simulink library "AeroLib"  (Simulink 6.0)
settings: Solver=ode45  SolverMode=SingleTasking  StartTime=0.0  StopTime=10.0  RelTol=1e-3
undefined symbols (not defined in the file): Aero, Ap, Atm, Control, Controls, Eng, Flight_cg, Flight_DamperON, Flight_delta_isa, Flight_DeltaSpiral, Flight_InertiaSelect, Flight_ixx, Flight_ixz, Flight_iyy, Flight_izz, Flight_latitude, Flight_LoiterLenght, Flight_LoiterMode, Flight_LoiterRadius, Flight_longitude, Flight_MaxTargetPoints, Flight_SensorsON, Flight_TimeStep, Flight_TowerWind_X, Flight_TowerWind_Y, Flight_TowerWind_Z, Flight_TowerWindON, Flight_Trimming, Flight_TurbON, Flight_weight, Flight_WindGustON, Flight_WindShearON, Flight_ycg, Flight_zcg, Geom, Lgear, Mass, PEG_CDwbnp, PEG_CLht, PEG_CLht_elev, PEG_CLwbnp, PEG_CMht, PEG_CMwbnp, PEG_CNbeta, PEG_CNr, PEG_CNrud, PEG_CRail, PEG_CRbeta, PEG_CRp, PEG_CRrud, PEG_CYbeta, PEG_CYrud, pow, Sensors
libraries: AeroLib x133, simulink3 x49, simulink x37, aerospace x11
(part 5 of 7)

== system AeroLib/GroundReactions/Landing_Gear/GHM Ground_Reactions ==
  MUeLmg : Inport  Port=1  LatchInput=off
  MUsLmg : Inport  Port=2  LatchInput=off
  FstrLmg : Inport  Port=3  LatchInput=off
  Rlmg : Inport  Port=4  LatchInput=off
  TireCompLmg : Inport  Port=5  LatchInput=off
  MUeNg : Inport  Port=6  LatchInput=off
  MUsNg : Inport  Port=7  LatchInput=off
  FstrNg : Inport  Port=8  LatchInput=off
  Rng : Inport  Port=9  LatchInput=off
  TireCompNg : Inport  Port=10  LatchInput=off
  NoseWheelAng : Inport  Port=11  LatchInput=off
  EulerRad : Inport  Port=12  LatchInput=off
  MUeRmg : Inport  Port=13  LatchInput=off
  MUsRmg : Inport  Port=14  LatchInput=off
  FstrRmg : Inport  Port=15  LatchInput=off
  Rrmg : Inport  Port=16  LatchInput=off
  TireCompRmg : Inport  Port=17  LatchInput=off
  Bus Creator : BusCreator  DialogController=Simulink.DDGSource_Bus  Inputs=9
  Demux : Demux  Outputs=3
  Demux1 : Demux  Outputs=3
  Moments : Subsystem
  Reactions1 : Subsystem
  GR_Out : Outport
  wires:
  MUeLmg/1 -> Reactions1/1(MUeLmg)
  MUsLmg/1 -> Reactions1/2(MUsLmg)
  FstrLmg/1 -> Reactions1/3(FstrLmg)
  EulerRad/1 -> Reactions1/10(EulerRad)  "DCbg"
  MUeNg/1 -> Reactions1/4(MUeNg)
  MUsNg/1 -> Reactions1/5(MUsNg)
  FstrNg/1 -> Reactions1/6(FstrNg)
  MUeRmg/1 -> Reactions1/7(MUeRmg)
  MUsRmg/1 -> Reactions1/8(MUsRmg)
  FstrRmg/1 -> Reactions1/9(FstrRmg)
  Reactions1/2(FgearLMG) -> Moments/1(FgearLmg)
  Reactions1/3(FgearNG) -> Moments/2(FgearNg)
  Reactions1/4(FgearRMG) -> Moments/3(FgearRmg)
  Rlmg/1 -> Moments/4(Rlmg)
  TireCompLmg/1 -> Bus Creator/7  "TireCompLmg"
  Rng/1 -> Moments/5(Rng)
  TireCompNg/1 -> Bus Creator/8  "TireCompNg"
  Rrmg/1 -> Moments/6(Rrmg)
  TireCompRmg/1 -> Bus Creator/9  "TireCompRmg"
  NoseWheelAng/1 -> Reactions1/11(NoseWheelAng)
  Bus Creator/1 -> GR_Out/1
  Reactions1/1(Fgear) -> Demux/1
  Demux/1 -> Bus Creator/1  "Xground"
  Demux/2 -> Bus Creator/2  "Yground"
  Demux/3 -> Bus Creator/3  "Zground"
  Moments/1(Mgear) -> Demux1/1
  Demux1/1 -> Bus Creator/4  "Lground"
  Demux1/2 -> Bus Creator/5  "Mground"
  Demux1/3 -> Bus Creator/6  "Nground"

== system AeroLib/GroundReactions/Landing_Gear/Left Main Gear Dynamics ==
  Brake : Inport  Port=1  LatchInput=off
  VelB : Inport  Port=2  LatchInput=off
  RatesB : Inport  Port=3  LatchInput=off
  DCbg : Inport  Port=4  LatchInput=off
  Hagl : Inport  Port=5  LatchInput=off
  Conf_Tire_RposLmg : Inport  Port=6  LatchInput=off
  Ground_Tire Contact : Subsystem
  Ground_Tire Friction : Subsystem
  LGEAR Accelerations : Subsystem
  LGEAR States : Subsystem
  MUeff : Outport
  MUside : Outport  Port=2
  TireForce : Outport  Port=3
  Rtb : Outport  Port=4
  TireComp : Outport  Port=5
  wires:
  Conf_Tire_RposLmg/1 -> Ground_Tire Contact/7(Conf_Tire_RposLmg)
  DCbg/1 -> Ground_Tire Contact/1(DCbg)
  Brake/1 -> Ground_Tire Friction/3(Brake)
  Ground_Tire Contact/2(Vtg) -> Ground_Tire Friction/2(Vtg)
  Ground_Tire Contact/1(Rtb) -> Rtb/1
  VelB/1 -> Ground_Tire Contact/2(VelB)
  RatesB/1 -> Ground_Tire Contact/3(RatesB)
  Ground_Tire Friction/2(MUeff) -> MUeff/1
  Ground_Tire Friction/1(MUside) -> MUside/1
  LGEAR States/1(Sdot) -> Ground_Tire Contact/4(Sdot), LGEAR Accelerations/2(Sdot)
  LGEAR States/2(S) -> Ground_Tire Contact/5(S), LGEAR Accelerations/3(S)
  LGEAR Accelerations/2(S2dot) -> LGEAR States/1(S2dot)
  LGEAR Accelerations/3(TireComp) -> Ground_Tire Contact/6(TireComp), TireComp/1
  Hagl/1 -> LGEAR Accelerations/1(Hagl)
  LGEAR Accelerations/1(TireForce) -> Ground_Tire Friction/1(TireForce), TireForce/1

== system AeroLib/GroundReactions/Landing_Gear/Nose Gear Dynamics ==
  VelB : Inport  Port=1  LatchInput=off
  RatesB : Inport  Port=2  LatchInput=off
  DCbg : Inport  Port=3  LatchInput=off
  Hagl : Inport  Port=4  LatchInput=off
  Conf_Tire_RposNg : Inport  Port=5  LatchInput=off
  Caster : Inport  Port=6  LatchInput=off
  NoseWheel : Inport  Port=7  LatchInput=off
  Ground_Tire Contact : Subsystem
  Ground_Tire Friction : Subsystem
  LGEAR Accelerations : Subsystem
  LGEAR States : Subsystem
  NoseWheelAngle : Subsystem
  MUeff : Outport
  MUside : Outport  Port=2
  TireForce : Outport  Port=3
  Rtb : Outport  Port=4
  TireComp : Outport  Port=5
  NoseWheelAng : Outport  Port=6
  wires:
  Conf_Tire_RposNg/1 -> Ground_Tire Contact/7(Conf_Tire_RposNg)
  LGEAR Accelerations/1(TireForce) -> TireForce/1, Ground_Tire Friction/1(TireForce)
  Hagl/1 -> LGEAR Accelerations/1(Hagl)
  LGEAR Accelerations/3(TireComp) -> Ground_Tire Contact/6(TireComp), TireComp/1
  LGEAR Accelerations/2(S2dot) -> LGEAR States/1(S2dot)
  LGEAR States/2(S) -> Ground_Tire Contact/5(S), LGEAR Accelerations/3(S)
  LGEAR States/1(Sdot) -> Ground_Tire Contact/4(Sdot), LGEAR Accelerations/2(Sdot)
  Ground_Tire Friction/1(MUside) -> MUside/1
  Ground_Tire Friction/2(MUeff) -> MUeff/1
  RatesB/1 -> Ground_Tire Contact/3(RatesB)
  VelB/1 -> Ground_Tire Contact/2(VelB)
  Ground_Tire Contact/1(Rtb) -> Rtb/1
  Ground_Tire Contact/2(Vtg) -> Ground_Tire Friction/2(Vtg), NoseWheelAngle/1(Vtg)
  DCbg/1 -> Ground_Tire Contact/1(DCbg)
  Caster/1 -> NoseWheelAngle/2(Caster)
  NoseWheel/1 -> NoseWheelAngle/3(NoseWheelAng)
  NoseWheelAngle/1(Out1) -> NoseWheelAng/1

== system AeroLib/GroundReactions/Landing_Gear/Right Main Gear Dynamics ==
  Brake : Inport  Port=1  LatchInput=off
  VelB : Inport  Port=2  LatchInput=off
  RatesB : Inport  Port=3  LatchInput=off
  DCbg : Inport  Port=4  LatchInput=off
  Hagl : Inport  Port=5  LatchInput=off
  Conf_Tire_RposRmg : Inport  Port=6  LatchInput=off
  Ground_Tire Contact : Subsystem
  Ground_Tire Friction : Subsystem
  LGEAR Accelerations : Subsystem
  LGEAR States : Subsystem
  MUeff : Outport
  MUside : Outport  Port=2
  TireForce : Outport  Port=3
  Rtb : Outport  Port=4
  TireComp : Outport  Port=5
  wires:
  LGEAR Accelerations/3(TireComp) -> TireComp/1, Ground_Tire Contact/6(TireComp)
  LGEAR Accelerations/2(S2dot) -> LGEAR States/1(S2dot)
  Conf_Tire_RposRmg/1 -> Ground_Tire Contact/7(Conf_Tire_RposRmg)
  DCbg/1 -> Ground_Tire Contact/1(DCbg)
  Brake/1 -> Ground_Tire Friction/3(Brake)
  Ground_Tire Contact/2(Vtg) -> Ground_Tire Friction/2(Vtg)
  Ground_Tire Contact/1(Rtb) -> Rtb/1
  VelB/1 -> Ground_Tire Contact/2(VelB)
  RatesB/1 -> Ground_Tire Contact/3(RatesB)
  Ground_Tire Friction/2(MUeff) -> MUeff/1
  Ground_Tire Friction/1(MUside) -> MUside/1
  LGEAR States/1(Sdot) -> LGEAR Accelerations/2(Sdot), Ground_Tire Contact/4(Sdot)
  LGEAR States/2(S) -> LGEAR Accelerations/3(S), Ground_Tire Contact/5(S)
  Hagl/1 -> LGEAR Accelerations/1(Hagl)
  LGEAR Accelerations/1(TireForce) -> Ground_Tire Friction/1(TireForce), TireForce/1

== system AeroLib/Propulsion/Booster/Fthrust_Booster ==
  LH NT : Inport  Port=1  LatchInput=off
  Constant : Constant  Value=0
  Fcn : Fcn  Expr=u*cos(pitch*pi/180)
  Fcn2 : Fcn  Expr=-u*sin(pitch*pi/180)
  Mux : Mux  Inputs=3
  LHFthr : Outport
  wires:
  Mux/1 -> LHFthr/1
  Fcn2/1 -> Mux/3
  Constant/1 -> Mux/2
  Fcn/1 -> Mux/1
  LH NT/1 -> Fcn/1, Fcn2/1

== system AeroLib/Propulsion/Booster/Thrust ==
  In1 : Inport  Port=1  LatchInput=off
  From_Reset : Inport  Port=2  LatchInput=off
  Constant : Constant  Value=0
  Gain_Amp : Gain  Gain=10  SaturateOnIntegerOverflow=on
  Stateless_Integrator : AeroLib/AMS_StatelessFilters/Stateless_Integrator
  Sum : Sum  Inputs=|+-  SaturateOnIntegerOverflow=on  InputSameDT=on
  Out1 : Outport
  wires:
  Sum/1 -> Gain_Amp/1  "err"
  Stateless_Integrator/1 -> Sum/2, Out1/1  "Stab"
  Gain_Amp/1 -> Stateless_Integrator/3
  In1/1 -> Sum/1
  Constant/1 -> Stateless_Integrator/2
  From_Reset/1 -> Stateless_Integrator/1

== system AeroLib/Propulsion/Engine_Transient/Engine_Transient_LH ==
  Throttle : Inport  Port=1  LatchInput=off
  From_Reset : Inport  Port=2  LatchInput=off
  Max : Constant  Value=Eng.MaxThrottle
  Min : Constant  Value=Eng.MinThrottle
  SpoolUpFreq : Gain  Gain=0.02  SaturateOnIntegerOverflow=on
  Stateless_LimIntegrator : AeroLib/AMS_StatelessFilters/Stateless_LimIntegrator
  Sum : Sum  Inputs=|+-  SaturateOnIntegerOverflow=on  InputSameDT=on
  TLA : Outport
  wires:
  SpoolUpFreq/1 -> Stateless_LimIntegrator/3
  Sum/1 -> SpoolUpFreq/1
  Stateless_LimIntegrator/1 -> Sum/2, TLA/1
  Throttle/1 -> Sum/1, Stateless_LimIntegrator/2
  Max/1 -> Stateless_LimIntegrator/5
  Min/1 -> Stateless_LimIntegrator/4
  From_Reset/1 -> Stateless_LimIntegrator/1

== system AeroLib/Propulsion/Engine_Transient/Engine_Transient_RH ==
  Throttle : Inport  Port=1  LatchInput=off
  From_Reset : Inport  Port=2  LatchInput=off
  Max : Constant  Value=Eng.MaxThrottle
  Min : Constant  Value=Eng.MinThrottle
  SpoolUpFreq : Gain  Gain=0.02  SaturateOnIntegerOverflow=on
  Stateless_LimIntegrator : AeroLib/AMS_StatelessFilters/Stateless_LimIntegrator
  Sum : Sum  Inputs=|+-  SaturateOnIntegerOverflow=on  InputSameDT=on
  TLA : Outport
  wires:
  From_Reset/1 -> Stateless_LimIntegrator/1
  Min/1 -> Stateless_LimIntegrator/4
  Max/1 -> Stateless_LimIntegrator/5
  Throttle/1 -> Stateless_LimIntegrator/2, Sum/1
  Stateless_LimIntegrator/1 -> TLA/1, Sum/2
  Sum/1 -> SpoolUpFreq/1
  SpoolUpFreq/1 -> Stateless_LimIntegrator/3

== system AeroLib/Propulsion/Fixed_Pitch_Propeller/Mach_Number_Effect ==
  J : Inport  Port=1  LatchInput=off
  Prop_rps : Inport  Port=2  LatchInput=off
  TAS : Inport  Port=3  LatchInput=off
  Mach : Inport  Port=4  LatchInput=off
  CP_coef : simulink/Lookup Tables/Interpolation (n-D) using PreLookup  numDimsPopupSelect=2  explicitNumDims=2  table=Eng.Prop.Kcp'  interpMethod=Linear  extrapMethod=Linear  rangeErrorMode=None  NumSelectionDims=0
  Constant : Constant  Value=0.75*pi
  Constant1 : Constant  Value=Eng.Prop.Twist
  Gain2 : Gain  Gain=180/pi  SaturateOnIntegerOverflow=on
  Km_coef : simulink/Lookup Tables/Interpolation (n-D) using PreLookup  numDimsPopupSelect=2  explicitNumDims=2  table=Eng.Prop.Kct'  interpMethod=Linear  extrapMethod=Linear  rangeErrorMode=None  NumSelectionDims=0
  Mach_Propeller : Fcn  Expr=sqrt( u(2)^2 + (pi*u(1)*Eng.Prop.diam)^2)/u(3)
  Mux2 : Mux  Inputs=3
  PreLook-Up Index Search : simulink/Lookup Tables/PreLookup Index Search  bpData=Eng.Prop.alp  searchMode=Binary Search  cacheBpFlag=off  outputFlag=off  IndexDataType=uint32  extrapMode=Linear Extrapolation  rangeErrorMode=None
  PreLook-Up Index Search1 : simulink/Lookup Tables/PreLookup Index Search  bpData=Eng.Prop.Mr  searchMode=Binary Search  cacheBpFlag=off  outputFlag=off  IndexDataType=uint32  extrapMode=Linear Extrapolation  rangeErrorMode=None
  Product2 : Product  Inputs=*/  SaturateOnIntegerOverflow=on  InputSameDT=on
  Product3 : Product  Inputs=*/  SaturateOnIntegerOverflow=on  InputSameDT=on
  Saturation : Saturate  UpperLimit=1.7  LowerLimit=1
  Saturation1 : Saturate  UpperLimit=1  LowerLimit=0.8
  Sum : Sum  Inputs=|-+  SaturateOnIntegerOverflow=on  InputSameDT=on
  Trigonometric Function : Trigonometry  Operator=atan
  Km : Outport
  Kcp : Outport  Port=2
  wires:
  Mux2/1 -> Mach_Propeller/1
  Product2/1 -> Mux2/3
  CP_coef/1 -> Saturation/1
  Sum/1 -> PreLook-Up Index Search/1
  Constant1/1 -> Sum/2
  Gain2/1 -> Sum/1
  Mach_Propeller/1 -> PreLook-Up Index Search1/1
  PreLook-Up Index Search/1 -> CP_coef/2, Km_coef/2
  PreLook-Up Index Search1/1 -> CP_coef/1, Km_coef/1
  Trigonometric Function/1 -> Gain2/1
  Product3/1 -> Trigonometric Function/1
  Constant/1 -> Product3/2
  Prop_rps/1 -> Mux2/1
  TAS/1 -> Mux2/2, Product2/1
  J/1 -> Product3/1
  Saturation/1 -> Kcp/1
  Mach/1 -> Product2/2
  Km_coef/1 -> Saturation1/1
  Saturation1/1 -> Km/1

== system AeroLib/Propulsion/Jet_Engine/Engine_Tables ==
  TRA : Inport  Port=1  LatchInput=off
  Mach : Inport  Port=2  LatchInput=off
  Alt : Inport  Port=3  LatchInput=off
  From_Reset : Inport  Port=4  LatchInput=off
  FuelCut : Inport  Port=5  LatchInput=off
  Constant1 : Constant  Value=0
  Constant5 : Constant  Value=0
  Constant6 : Constant  Value=Eng.Fuel.mass
  Fcn1 : Fcn  Expr=u(2)*(1-u(1))
  Fcn2 : Fcn  Expr=u(1)*(1-u(2))
  Fcn3 : Fcn  Expr=1-u
  FuelDensity : Gain  Gain=0.7  SaturateOnIntegerOverflow=on
  Fuel_Flow : simulink/Lookup Tables/Interpolation (n-D) using PreLookup  numDimsPopupSelect=1  explicitNumDims=2  table=Eng.Cons  interpMethod=Linear  extrapMethod=Linear  rangeErrorMode=None  NumSelectionDims=0
  Gross_Thrust : simulink/Lookup Tables/Interpolation (n-D) using PreLookup  numDimsPopupSelect=3  explicitNumDims=2  table=Eng.GrossThrust  interpMethod=Linear  extrapMethod=Linear  rangeErrorMode=None  NumSelectionDims=0
  Mux : Mux  Inputs=2
  Mux1 : Mux  Inputs=2
  PreLook-Up Index Search : simulink/Lookup Tables/PreLookup Index Search  bpData=Eng.Mach  searchMode=Binary Search  cacheBpFlag=off  outputFlag=off  IndexDataType=uint32  extrapMode=Linear Extrapolation  rangeErrorMode=None
  PreLook-Up Index Search1 : simulink/Lookup Tables/PreLookup Index Search  bpData=Eng.Alt  searchMode=Binary Search  cacheBpFlag=off  outputFlag=off  IndexDataType=uint32  extrapMode=Linear Extrapolation  rangeErrorMode=None
  PreLook-Up Index Search2 : simulink/Lookup Tables/PreLookup Index Search  bpData=Eng.Throttle  searchMode=Binary Search  cacheBpFlag=off  outputFlag=off  IndexDataType=uint32  extrapMode=Linear Extrapolation  rangeErrorMode=None
  Product : Product  SaturateOnIntegerOverflow=on  InputSameDT=on
  Ram_Drag : simulink/Lookup Tables/Interpolation (n-D) using PreLookup  numDimsPopupSelect=3  explicitNumDims=2  table=Eng.RamDrag  interpMethod=Linear  extrapMethod=Linear  rangeErrorMode=None  NumSelectionDims=0
  Stateless_LimIntegrator : AeroLib/AMS_StatelessFilters/Stateless_LimIntegrator
  Sum1 : Sum  Inputs=+-  SaturateOnIntegerOverflow=on  InputSameDT=on
  GrossThrust : Outport
  NetThrust : Outport  Port=2
  RamDrag : Outport  Port=3
  Fuel_Mass : Outport  Port=4
  wires:
  Fuel_Flow/1 -> Product/1
  Product/1 -> FuelDensity/1
  Fcn3/1 -> Product/2
  Sum1/1 -> NetThrust/1  "NetThrust"
  Alt/1 -> PreLook-Up Index Search1/1
  Mach/1 -> PreLook-Up Index Search/1
  TRA/1 -> PreLook-Up Index Search2/1
  Ram_Drag/1 -> Mux/2  "RamDrag"
  PreLook-Up Index Search2/1 -> Fuel_Flow/1, Ram_Drag/1, Gross_Thrust/1
  PreLook-Up Index Search1/1 -> Ram_Drag/3, Gross_Thrust/3
  PreLook-Up Index Search/1 -> Ram_Drag/2, Gross_Thrust/2
  Fcn1/1 -> RamDrag/1, Sum1/2  "RamDrag"
  FuelCut/1 -> Fcn3/1, Mux/1, Mux1/2
  Mux/1 -> Fcn1/1
  Fcn2/1 -> GrossThrust/1, Sum1/1  "GrossThrust"
  Gross_Thrust/1 -> Mux1/1  "GrossThrust"
  Mux1/1 -> Fcn2/1
  FuelDensity/1 -> Stateless_LimIntegrator/3
  Constant1/1 -> Stateless_LimIntegrator/2
  From_Reset/1 -> Stateless_LimIntegrator/1
  Constant5/1 -> Stateless_LimIntegrator/4
  Constant6/1 -> Stateless_LimIntegrator/5
  Stateless_LimIntegrator/1 -> Fuel_Mass/1

== system AeroLib/Propulsion/Piston_Engine_Propeller/Power_Limit ==
  Avail_Power : Inport  Port=1  LatchInput=off
  Rpm : Inport  Port=2  LatchInput=off
  Power_Demand : Inport  Port=3  LatchInput=off
  Fcn1 : Fcn  Expr=u >= 0
  Fcn2 : Fcn  Expr=u(1) - u(2)
  Fcn4 : Fcn  Expr=u < 0
  Gain : Gain  Orientation=left  Gain=5  SaturateOnIntegerOverflow=on
  Memory2 : Memory  Orientation=left
  Mux1 : Mux  Inputs=2
  Product1 : Product  SaturateOnIntegerOverflow=on  InputSameDT=on
  Rpm_Limit : Subsystem
  Sum1 : Sum  Orientation=left  Inputs=+++  SaturateOnIntegerOverflow=on  InputSameDT=on
  Switch : Switch  Threshold=0.5  SaturateOnIntegerOverflow=on  InputSameDT=on
  Delta_Rpm : Outport  Orientation=left
  wires:
  Gain/1 -> Delta_Rpm/1
  Switch/1 -> Sum1/3
  Rpm_Limit/1(Rpm_Command) -> Sum1/2
  Rpm/1 -> Rpm_Limit/2(Rpm)
  Power_Demand/1 -> Mux1/2
  Avail_Power/1 -> Mux1/1
  Product1/1 -> Switch/1
  Fcn4/1 -> Product1/1
  Memory2/1 -> Gain/1, Fcn4/1, Sum1/1
  Sum1/1 -> Memory2/1
  Mux1/1 -> Fcn2/1
  Fcn1/1 -> Switch/2
  Fcn2/1 -> Rpm_Limit/1(deltaPower), Switch/3, Product1/2, Fcn1/1

== system AeroLib/Propulsion/Thrust_Components/LH_Fthrust ==
  LH NT : Inport  Port=1  LatchInput=off
  Fcn : Fcn  Expr=u*cos(pitch)*cos(toeout)
  Fcn1 : Fcn  Expr=-u*sin(toeout)
  Fcn2 : Fcn  Expr=-u*sin(pitch)
  Mux : Mux  Inputs=3
  LHFthr : Outport
  wires:
  Mux/1 -> LHFthr/1
  Fcn2/1 -> Mux/3
  Fcn1/1 -> Mux/2
  Fcn/1 -> Mux/1
  LH NT/1 -> Fcn2/1, Fcn1/1, Fcn/1

== system AeroLib/Propulsion/Thrust_Components/RH_Fthrust ==
  RH NT : Inport  Port=1  LatchInput=off
  Fcn : Fcn  Expr=u*cos(pitch)*cos(toeout)
  Fcn1 : Fcn  Expr=u*sin(toeout)
  Fcn2 : Fcn  Expr=-u*sin(pitch)
  Mux : Mux  Inputs=3
  RHFthr : Outport
  wires:
  RH NT/1 -> Fcn/1, Fcn1/1, Fcn2/1
  Fcn/1 -> Mux/1
  Fcn1/1 -> Mux/2
  Fcn2/1 -> Mux/3
  Mux/1 -> RHFthr/1

== system AeroLib/Propulsion/Variable_Pitch_Propeller/Mach_Number_Effect ==
  J : Inport  Port=1  LatchInput=off
  Prop_rps : Inport  Port=2  LatchInput=off
  TAS : Inport  Port=3  LatchInput=off
  Mach : Inport  Port=4  LatchInput=off
  Prop_Pitch_deg : Inport  Port=5  LatchInput=off
  CP_coef : simulink/Lookup Tables/Interpolation (n-D) using PreLookup  numDimsPopupSelect=2  explicitNumDims=2  table=Eng.Prop.Kcp'  interpMethod=Linear  extrapMethod=Linear  rangeErrorMode=None  NumSelectionDims=0
  Constant : Constant  Value=0.75*pi
  Gain2 : Gain  Gain=180/pi  SaturateOnIntegerOverflow=on
  Km_coef : simulink/Lookup Tables/Interpolation (n-D) using PreLookup  numDimsPopupSelect=2  explicitNumDims=2  table=Eng.Prop.Kct'  interpMethod=Linear  extrapMethod=Linear  rangeErrorMode=None  NumSelectionDims=0
  Mach_Propeller : Fcn  Expr=sqrt( u(2)^2 + (pi*u(1)*Eng.Prop.diam)^2)/u(3)
  Mux2 : Mux  Inputs=3
  PreLook-Up Index Search : simulink/Lookup Tables/PreLookup Index Search  bpData=Eng.Prop.alp  searchMode=Binary Search  cacheBpFlag=off  outputFlag=off  IndexDataType=uint32  extrapMode=Linear Extrapolation  rangeErrorMode=None
  PreLook-Up Index Search1 : simulink/Lookup Tables/PreLookup Index Search  bpData=Eng.Prop.Mr  searchMode=Binary Search  cacheBpFlag=off  outputFlag=off  IndexDataType=uint32  extrapMode=Linear Extrapolation  rangeErrorMode=None
  Product2 : Product  Inputs=*/  SaturateOnIntegerOverflow=on  InputSameDT=on
  Product3 : Product  Inputs=*/  SaturateOnIntegerOverflow=on  InputSameDT=on
  Saturation : Saturate  UpperLimit=1.7  LowerLimit=1
  Saturation1 : Saturate  UpperLimit=1  LowerLimit=0.8
  Sum : Sum  Inputs=|-+  SaturateOnIntegerOverflow=on  InputSameDT=on
  Trigonometric Function : Trigonometry  Operator=atan
  Km : Outport
  Kcp : Outport  Port=2
  wires:
  Mux2/1 -> Mach_Propeller/1
  Product2/1 -> Mux2/3
  CP_coef/1 -> Saturation/1
  Sum/1 -> PreLook-Up Index Search/1
  Prop_Pitch_deg/1 -> Sum/2
  Gain2/1 -> Sum/1
  Mach_Propeller/1 -> PreLook-Up Index Search1/1
  PreLook-Up Index Search/1 -> CP_coef/2, Km_coef/2
  PreLook-Up Index Search1/1 -> CP_coef/1, Km_coef/1
  Trigonometric Function/1 -> Gain2/1
  Product3/1 -> Trigonometric Function/1
  Constant/1 -> Product3/2
  Prop_rps/1 -> Mux2/1
  TAS/1 -> Mux2/2, Product2/1
  J/1 -> Product3/1
  Saturation/1 -> Kcp/1
  Mach/1 -> Product2/2
  Km_coef/1 -> Saturation1/1
  Saturation1/1 -> Km/1

== system AeroLib/Sensors/Air_Data_Computer/SensorsOFF ==
  Clock : Clock
      settings: Decimation=10
  Constant1 : Constant  Value=Flight_SensorsON
  Fcn : Fcn  Expr=u <= 0+eps
  or : Logic  Operator=OR
  or1 : Logic  Operator=NOT
  SensorsOFF : Outport
  wires:
  Clock/1 -> Fcn/1
  Constant1/1 -> or1/1  "DT"
  Fcn/1 -> or/2
  or/1 -> SensorsOFF/1
  or1/1 -> or/1

== system AeroLib/Sensors/Global_Positioning_System/SensorsOFF ==
  Clock : Clock
      settings: Decimation=10
  Constant1 : Constant  Value=Flight_SensorsON
  Fcn : Fcn  Expr=u <= 0+eps
  or : Logic  Operator=OR
  or1 : Logic  Operator=NOT
  SensorsOFF : Outport
  wires:
  or1/1 -> or/1
  or/1 -> SensorsOFF/1
  Fcn/1 -> or/2
  Constant1/1 -> or1/1  "DT"
  Clock/1 -> Fcn/1

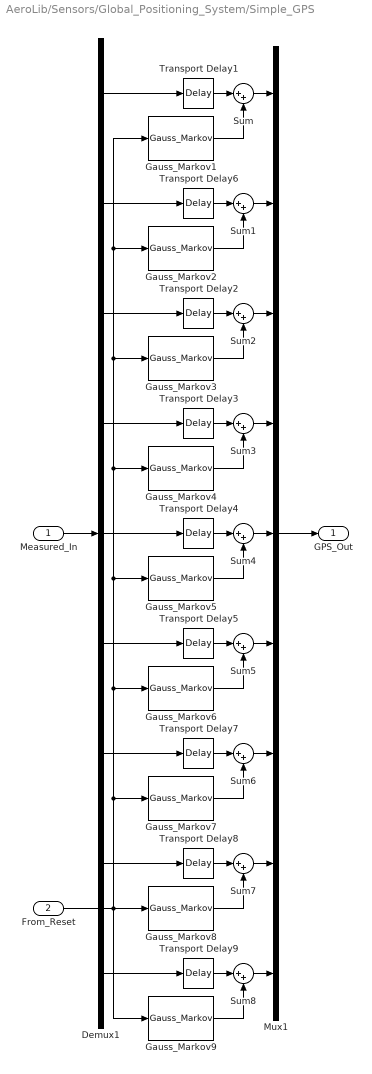
== system AeroLib/Sensors/Global_Positioning_System/Simple_GPS ==
  Measured_In : Inport  Port=1  LatchInput=off
  "From_Reset " : Inport  Port=2  LatchInput=off
  Demux1 : Demux  Outputs=9
  Gauss_Markov1 : AeroLib/Sensors/Gauss_Markov  Seed=Seed(1)  tau=Time(1)  Var=Var(1)
  Gauss_Markov2 : AeroLib/Sensors/Gauss_Markov  Seed=Seed(2)  tau=Time(2)  Var=Var(2)
  Gauss_Markov3 : AeroLib/Sensors/Gauss_Markov  Seed=Seed(3)  tau=Time(3)  Var=Var(3)
  Gauss_Markov4 : AeroLib/Sensors/Gauss_Markov  Seed=Seed(4)  tau=Time(4)  Var=Var(4)
  Gauss_Markov5 : AeroLib/Sensors/Gauss_Markov  Seed=Seed(5)  tau=Time(5)  Var=Var(5)
  Gauss_Markov6 : AeroLib/Sensors/Gauss_Markov  Seed=Seed(6)  tau=Time(6)  Var=Var(6)
  Gauss_Markov7 : AeroLib/Sensors/Gauss_Markov  Seed=Seed(7)  tau=Time(7)  Var=Var(7)
  Gauss_Markov8 : AeroLib/Sensors/Gauss_Markov  Seed=Seed(8)  tau=Time(8)  Var=Var(8)
  Gauss_Markov9 : AeroLib/Sensors/Gauss_Markov  Seed=Seed(9)  tau=Time(9)  Var=Var(9)
  Mux1 : Mux  Inputs=9
  Sum{,1..8} (9 alike) : Sum  Inputs=|++  SaturateOnIntegerOverflow=on  InputSameDT=on
  Transport Delay1 : TransportDelay  DelayTime=Time_delay(1)
  Transport Delay2 : TransportDelay  DelayTime=Time_delay(3)
  Transport Delay3 : TransportDelay  DelayTime=Time_delay(4)
  Transport Delay4 : TransportDelay  DelayTime=Time_delay(5)
  Transport Delay5 : TransportDelay  DelayTime=Time_delay(6)
  Transport Delay6 : TransportDelay  DelayTime=Time_delay(2)
  Transport Delay7 : TransportDelay  DelayTime=Time_delay(7)
  Transport Delay8 : TransportDelay  DelayTime=Time_delay(8)
  Transport Delay9 : TransportDelay  DelayTime=Time_delay(9)
  GPS_Out : Outport
  wires:
  Mux1/1 -> GPS_Out/1
  Measured_In/1 -> Demux1/1
  Gauss_Markov1/1 -> Sum/2
  Transport Delay1/1 -> Sum/1
  Gauss_Markov2/1 -> Sum1/2
  Transport Delay6/1 -> Sum1/1
  Gauss_Markov3/1 -> Sum2/2
  Transport Delay2/1 -> Sum2/1
  Gauss_Markov4/1 -> Sum3/2
  Transport Delay3/1 -> Sum3/1
  Gauss_Markov5/1 -> Sum4/2
  Transport Delay4/1 -> Sum4/1
  Demux1/2 -> Transport Delay6/1
  Demux1/3 -> Transport Delay2/1
  Sum1/1 -> Mux1/2
  Demux1/4 -> Transport Delay3/1
  Sum3/1 -> Mux1/4
  Sum4/1 -> Mux1/5
  Demux1/5 -> Transport Delay4/1
  Gauss_Markov6/1 -> Sum5/2
  Transport Delay5/1 -> Sum5/1
  Sum5/1 -> Mux1/6
  Demux1/6 -> Transport Delay5/1
  Sum2/1 -> Mux1/3
  Demux1/1 -> Transport Delay1/1
  Sum/1 -> Mux1/1
  Gauss_Markov7/1 -> Sum6/2
  Transport Delay7/1 -> Sum6/1
  Sum6/1 -> Mux1/7
  Demux1/7 -> Transport Delay7/1
  Gauss_Markov8/1 -> Sum7/2
  Transport Delay8/1 -> Sum7/1
  Sum7/1 -> Mux1/8
  Demux1/8 -> Transport Delay8/1
  "From_Reset "/1 -> Gauss_Markov9/1, Gauss_Markov7/1, Gauss_Markov6/1, Gauss_Markov5/1, Gauss_Markov4/1, Gauss_Markov3/1, Gauss_Markov2/1, Gauss_Markov1/1, Gauss_Markov8/1
  Gauss_Markov9/1 -> Sum8/2
  Transport Delay9/1 -> Sum8/1
  Demux1/9 -> Transport Delay9/1
  Sum8/1 -> Mux1/9

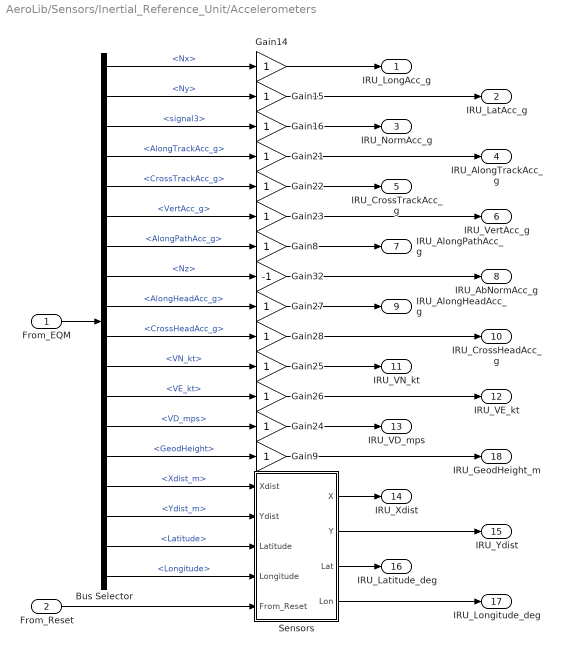
== system AeroLib/Sensors/Inertial_Reference_Unit/Accelerometers ==
  From_EQM : Inport  Port=1  LatchInput=off
  From_Reset : Inport  Port=2  LatchInput=off
  Bus Selector : BusSelector  DialogController=Simulink.DDGSource_Bus  OutputSignals=Nx,Ny,AccB.signal3,AlongTrackAcc_g,CrossTrackAcc_g,VertAcc_g,AlongPathAcc_g,Nz,AlongHeadAcc_g,CrossHeadAcc_g,VN_kt,VE_kt,VD_mps,GeodHeight,Xdist_m,Ydist_m,Latitude,Longitude
  Gain{8..9,14..16,21..28} (13 alike) : Gain  SaturateOnIntegerOverflow=on
  Gain32 : Gain  Gain=-1  SaturateOnIntegerOverflow=on
  Sensors : Subsystem
  IRU_LongAcc_g : Outport
  IRU_LatAcc_g : Outport  Port=2
  IRU_NormAcc_g : Outport  Port=3
  IRU_AlongTrackAcc_g : Outport  Port=4
  IRU_CrossTrackAcc_g : Outport  Port=5
  IRU_VertAcc_g : Outport  Port=6
  IRU_AlongPathAcc_g : Outport  Port=7
  IRU_AbNormAcc_g : Outport  Port=8
  IRU_AlongHeadAcc_g : Outport  Port=9
  IRU_CrossHeadAcc_g : Outport  Port=10
  IRU_VN_kt : Outport  Port=11
  IRU_VE_kt : Outport  Port=12
  IRU_VD_mps : Outport  Port=13
  IRU_Xdist : Outport  Port=14
  IRU_Ydist : Outport  Port=15
  IRU_Latitude_deg : Outport  Port=16
  IRU_Longitude_deg : Outport  Port=17
  IRU_GeodHeight_m : Outport  Port=18
  wires:
  From_Reset/1 -> Sensors/5(From_Reset)
  Bus Selector/14 -> Gain9/1  "<GeodHeight>"
  Gain9/1 -> IRU_GeodHeight_m/1
  Bus Selector/18 -> Sensors/4(Longitude)  "<Longitude>"
  Sensors/4(Lon) -> IRU_Longitude_deg/1
  Sensors/3(Lat) -> IRU_Latitude_deg/1
  Bus Selector/16 -> Sensors/2(Ydist)  "<Ydist_m>"
  Bus Selector/15 -> Sensors/1(Xdist)  "<Xdist_m>"
  Bus Selector/17 -> Sensors/3(Latitude)  "<Latitude>"
  Sensors/1(X) -> IRU_Xdist/1
  Sensors/2(Y) -> IRU_Ydist/1
  Bus Selector/13 -> Gain24/1  "<VD_mps>"
  Bus Selector/12 -> Gain26/1  "<VE_kt>"
  Bus Selector/11 -> Gain25/1  "<VN_kt>"
  Bus Selector/10 -> Gain28/1  "<CrossHeadAcc_g>"
  Bus Selector/9 -> Gain27/1  "<AlongHeadAcc_g>"
  Bus Selector/8 -> Gain32/1  "<Nz>"
  Bus Selector/7 -> Gain8/1  "<AlongPathAcc_g>"
  Bus Selector/6 -> Gain23/1  "<VertAcc_g>"
  Bus Selector/5 -> Gain22/1  "<CrossTrackAcc_g>"
  Bus Selector/4 -> Gain21/1  "<AlongTrackAcc_g>"
  Bus Selector/3 -> Gain16/1  "<signal3>"
  Bus Selector/2 -> Gain15/1  "<Ny>"
  Bus Selector/1 -> Gain14/1  "<Nx>"
  Gain24/1 -> IRU_VD_mps/1
  Gain25/1 -> IRU_VN_kt/1
  Gain26/1 -> IRU_VE_kt/1
  Gain27/1 -> IRU_AlongHeadAcc_g/1
  Gain28/1 -> IRU_CrossHeadAcc_g/1
  Gain32/1 -> IRU_AbNormAcc_g/1
  Gain8/1 -> IRU_AlongPathAcc_g/1
  Gain23/1 -> IRU_VertAcc_g/1
  Gain21/1 -> IRU_AlongTrackAcc_g/1
  Gain22/1 -> IRU_CrossTrackAcc_g/1
  Gain14/1 -> IRU_LongAcc_g/1
  Gain15/1 -> IRU_LatAcc_g/1
  Gain16/1 -> IRU_NormAcc_g/1
  From_EQM/1 -> Bus Selector/1

== system AeroLib/Sensors/Inertial_Reference_Unit/Airspeed_Detectors ==
  From_EQM : Inport  Port=1  LatchInput=off
  From_Atmos : Inport  Port=2  LatchInput=off
  From_Reset : Inport  Port=3  LatchInput=off
  Bus Selector : BusSelector  DialogController=Simulink.DDGSource_Bus  OutputSignals=GroundSpeed_kt
  Bus Selector1 : BusSelector  DialogController=Simulink.DDGSource_Bus  OutputSignals=KIAS,TAS_kt
  Constant : Constant
  Demux : Demux  Outputs=3
  MinMax : MinMax  Function=max  Inputs=2  SaturateOnIntegerOverflow=on  InputSameDT=on
  Mux : Mux  Inputs=3
  SensorsOFF : Subsystem
  Simple_Sensor : AeroLib/Sensors/Simple_Sensor  Var=Sensors.IRU.Speed.Var  Seed=Sensors.IRU.Speed.Seed  Max=600  Min=0  Time_Const=Sensors.IRU.Speed.TimeConst
  Switch : Switch  Threshold=0.5  SaturateOnIntegerOverflow=on  InputSameDT=on
  IRU_GrSpeed_kt : Outport
  IRU_KIAS : Outport  Port=2
  IRU_TAS_kt : Outport  Port=3
  wires:
  Simple_Sensor/1 -> Switch/3
  From_Reset/1 -> Simple_Sensor/3
  Mux/1 -> Simple_Sensor/2, Switch/1, Simple_Sensor/1
  Demux/2 -> IRU_KIAS/1
  Demux/3 -> IRU_TAS_kt/1
  SensorsOFF/1(SensorsOFF) -> Switch/2
  Bus Selector1/2 -> Mux/3  "<TAS_kt>"
  Bus Selector1/1 -> Mux/2  "<KIAS>"
  Bus Selector/1 -> Mux/1  "<GroundSpeed_kt>"
  From_Atmos/1 -> Bus Selector1/1
  From_EQM/1 -> Bus Selector/1
  Demux/1 -> IRU_GrSpeed_kt/1
  Switch/1 -> MinMax/2
  MinMax/1 -> Demux/1
  Constant/1 -> MinMax/1

== system AeroLib/Sensors/Inertial_Reference_Unit/Altitude_Sensors ==
  From_Atmos : Inport  Port=1  LatchInput=off
  From_EQM : Inport  Port=2  LatchInput=off
  From_Reset : Inport  Port=3  LatchInput=off
  Bus Selector1 : BusSelector  DialogController=Simulink.DDGSource_Bus  OutputSignals=PresAlt_ft
  Bus Selector2 : BusSelector  DialogController=Simulink.DDGSource_Bus  OutputSignals=Hagl_ft
  SensorsOFF : Subsystem
  Simple_Sensor : AeroLib/Sensors/Simple_Sensor  Var=Sensors.IRU.Alt.Pres.Var  Seed=Sensors.IRU.Alt.Pres.Seed  Max=60000  Min=-500  Time_Const=Sensors.IRU.Alt.Pres.TimeConst
  Simple_Sensor1 : AeroLib/Sensors/Simple_Sensor  Var=Sensors.IRU.Alt.Radar.Var  Seed=Sensors.IRU.Alt.Radar.Seed  Max=3000  Min=0  Time_Const=Sensors.IRU.Alt.Radar.TimeConst
  Switch : Switch  Threshold=0.5  SaturateOnIntegerOverflow=on  InputSameDT=on
  Switch1 : Switch  Threshold=0.5  SaturateOnIntegerOverflow=on  InputSameDT=on
  IRU_PresAlt_ft : Outport
  IRU_RadarAlt_ft : Outport  Port=2
  wires:
  From_Reset/1 -> Simple_Sensor1/3, Simple_Sensor/3
  Simple_Sensor1/1 -> Switch1/3
  Simple_Sensor/1 -> Switch/3
  SensorsOFF/1(SensorsOFF) -> Switch1/2, Switch/2
  Bus Selector2/1 -> Simple_Sensor1/2, Switch1/1, Simple_Sensor1/1  "<Hagl_ft>"
  From_EQM/1 -> Bus Selector2/1
  From_Atmos/1 -> Bus Selector1/1
  Bus Selector1/1 -> Simple_Sensor/2, Switch/1, Simple_Sensor/1  "<PresAlt_ft>"
  Switch/1 -> IRU_PresAlt_ft/1
  Switch1/1 -> IRU_RadarAlt_ft/1

== system AeroLib/Sensors/Inertial_Reference_Unit/Flow_Incidence_Angle_Sensors ==
  From_Atmos : Inport  Port=1  LatchInput=off
  From_Reset : Inport  Port=2  LatchInput=off
  Bus Selector1 : BusSelector  DialogController=Simulink.DDGSource_Bus  OutputSignals=Alpha,Beta
  Demux : Demux  Outputs=2
  Mux : Mux  Inputs=2
  SensorsOFF : Subsystem
  Simple_Sensor : AeroLib/Sensors/Simple_Sensor  Var=Sensors.IRU.AlphaBeta.Var  Seed=Sensors.IRU.AlphaBeta.Seed  Max=30  Min=-30  Time_Const=Sensors.IRU.AlphaBeta.TimeConst
  Switch : Switch  Threshold=0.5  SaturateOnIntegerOverflow=on  InputSameDT=on
  IRU_Alpha : Outport
  IRU_Beta : Outport  Port=2
  wires:
  Simple_Sensor/1 -> Switch/3
  From_Reset/1 -> Simple_Sensor/3
  Mux/1 -> Simple_Sensor/2, Switch/1, Simple_Sensor/1
  Switch/1 -> Demux/1
  Demux/2 -> IRU_Beta/1
  Demux/1 -> IRU_Alpha/1
  SensorsOFF/1(SensorsOFF) -> Switch/2
  Bus Selector1/2 -> Mux/2  "<Beta>"
  Bus Selector1/1 -> Mux/1  "<Alpha>"
  From_Atmos/1 -> Bus Selector1/1

== system AeroLib/Sensors/Inertial_Reference_Unit/Gyrospopes ==
  From_EQM : Inport  Port=1  LatchInput=off
  Bus Selector : BusSelector  DialogController=Simulink.DDGSource_Bus  OutputSignals=Phi_deg,The_deg,P_deg,Q_deg,R_deg,Track_deg,Psi_deg,Gamma_deg
  Fcn : Fcn  Expr=u+MagDev
  Fcn1 : Fcn  Expr=u+MagDev
  Fcn2 : Fcn  Expr=u+PlatformDev
  Gain{3..7,9..10} (7 alike) : Gain  SaturateOnIntegerOverflow=on
  Pitch_Gyro : Gain  SaturateOnIntegerOverflow=on
  Pitch_Rate_Gyro : Gain  SaturateOnIntegerOverflow=on
  Roll_Gyro : Gain  SaturateOnIntegerOverflow=on
  Roll_Rate_Gyro : Gain  SaturateOnIntegerOverflow=on
  Sum : Sum  Inputs=+-|  SaturateOnIntegerOverflow=on  InputSameDT=on
  Yaw_Rate_Gyro : Gain  SaturateOnIntegerOverflow=on
  IRU_Theta_deg : Outport
  IRU_Phi_deg : Outport  Port=2
  IRU_Q_degps : Outport  Port=3
  IRU_P_degps : Outport  Port=4
  IRU_R_degps : Outport  Port=5
  IRU_Track_deg : Outport  Port=6
  IRU_Head_deg : Outport  Port=7
  IRU_TrackMag_deg : Outport  Port=8
  IRU_HeadMag_deg : Outport  Port=9
  IRU_DriftAngle_deg : Outport  Port=10
  IRU_PlatformHead_deg : Outport  Port=11
  IRU_FPath_deg : Outport  Port=12
  wires:
  Gain10/1 -> IRU_FPath_deg/1
  Gain9/1 -> IRU_PlatformHead_deg/1
  Gain7/1 -> IRU_DriftAngle_deg/1
  Gain6/1 -> IRU_HeadMag_deg/1
  Gain5/1 -> IRU_TrackMag_deg/1
  Gain4/1 -> IRU_Head_deg/1
  Gain3/1 -> IRU_Track_deg/1
  Bus Selector/6 -> Fcn/1, Gain3/1, Sum/1  "<Track_deg>"
  Bus Selector/8 -> Gain10/1  "<Gamma_deg>"
  Bus Selector/7 -> Fcn1/1, Gain4/1, Sum/2, Fcn2/1  "<Psi_deg>"
  Fcn/1 -> Gain5/1
  Fcn1/1 -> Gain6/1
  Sum/1 -> Gain7/1
  Fcn2/1 -> Gain9/1
  Bus Selector/4 -> Pitch_Rate_Gyro/1  "<Q_deg>"
  Pitch_Gyro/1 -> IRU_Theta_deg/1
  Roll_Gyro/1 -> IRU_Phi_deg/1
  Pitch_Rate_Gyro/1 -> IRU_Q_degps/1
  Roll_Rate_Gyro/1 -> IRU_P_degps/1
  Yaw_Rate_Gyro/1 -> IRU_R_degps/1
  Bus Selector/2 -> Pitch_Gyro/1  "<The_deg>"
  Bus Selector/1 -> Roll_Gyro/1  "<Phi_deg>"
  Bus Selector/3 -> Roll_Rate_Gyro/1  "<P_deg>"
  Bus Selector/5 -> Yaw_Rate_Gyro/1  "<R_deg>"
  From_EQM/1 -> Bus Selector/1

== system AeroLib/Aerodynamics/Aerodynamics_Generic/LIft/CL Tail ==
  From_Inputs : Inport  Port=1  LatchInput=off
  Epsilon : Inport  Port=2  LatchInput=off
  From_Atmos : Inport  Port=3  LatchInput=off
  From_EQM : Inport  Port=4  LatchInput=off
  Bus Selector : BusSelector  DialogController=Simulink.DDGSource_Bus  OutputSignals=Elev_deg,Stab_deg
  Bus Selector1 : BusSelector  DialogController=Simulink.DDGSource_Bus  OutputSignals=Alpha,TAS,AlphaDot
  Bus Selector2 : BusSelector  DialogController=Simulink.DDGSource_Bus  OutputSignals=Q_rad
  Fcn1 : Fcn  Expr=u(1)+u(2)-u(3)+u(4)
  Fcn3 : Fcn  Expr=Geom.Htail.lt/u(1)*180/pi*(1.2*u(3)+0.32*u(2))
  Fcn5 : Fcn  Expr=(Aero.a1_deg*u(2) )*Geom.Htail.st/Geom.Wing.sw
  Fcn6 : Fcn  Expr=( Aero.a2_deg*u(1))*Geom.Htail.st/Geom.Wing.sw
  Gain : Gain  Gain=PEG_CLht  SaturateOnIntegerOverflow=on
  Gain1 : Gain  Gain=PEG_CLht_elev  SaturateOnIntegerOverflow=on
  Mux : Mux  Inputs=3
  Mux1 : Mux
  Mux2 : Mux  Inputs=2
  Sum : Sum  Inputs=|++  SaturateOnIntegerOverflow=on  InputSameDT=on
  CL_Tail : Outport
  wires:
  Gain1/1 -> Sum/2
  Gain/1 -> Sum/1
  Fcn6/1 -> Gain1/1
  Fcn5/1 -> Gain/1  "CL_Tail"
  Sum/1 -> CL_Tail/1
  Bus Selector/1 -> Mux2/1  "<Elev_deg>"
  Fcn3/1 -> Mux1/4
  Bus Selector1/3 -> Mux/2  "<AlphaDot>"
  From_Inputs/1 -> Bus Selector/1
  From_Atmos/1 -> Bus Selector1/1
  From_EQM/1 -> Bus Selector2/1
  Bus Selector1/1 -> Mux1/2  "<Alpha>"
  Bus Selector1/2 -> Mux/1  "<TAS>"
  Bus Selector/2 -> Mux1/1  "<Stab_deg>"
  Bus Selector2/1 -> Mux/3  "<Q_rad>"
  Mux/1 -> Fcn3/1
  Fcn1/1 -> Mux2/2  "alpha_ht"
  Mux1/1 -> Fcn1/1
  Mux2/1 -> Fcn6/1, Fcn5/1
  Epsilon/1 -> Mux1/3  "Epsilon"

== system AeroLib/Aerodynamics/Aerodynamics_Pioneer/Aero Total/Stab2Body ==
  Alpha_Deg : Inport  Port=1  LatchInput=off
  Stab_Axis : Inport  Port=2  LatchInput=off
  Constant{1..2,4..5} (4 alike) : Constant  Value=0
  Constant3 : Constant
  Deg-->Rad : Gain  Gain=pi/180  SaturateOnIntegerOverflow=on
  Deg-->Rad1 : Gain  Gain=-1  SaturateOnIntegerOverflow=on
  Deg-->Rad2 : Gain  Gain=-1  SaturateOnIntegerOverflow=on
  Deg-->Rad3 : Gain  Gain=-1  SaturateOnIntegerOverflow=on
  Mux : Mux  Inputs=9
  Product : Product  Multiplication=Matrix(*)  SaturateOnIntegerOverflow=on  InputSameDT=on
  Reshape : simulink3/Signals & Systems/Reshape  OutputDimensionality=Customize  OutputDimensions=[3,3]
  Trigonometric Function : Trigonometry  Operator=cos
  Trigonometric Function2 : Trigonometry
  Trigonometric Function3 : Trigonometry  Operator=cos
  Trigonometric Function4 : Trigonometry
  Body_Axis : Outport
  wires:
  Deg-->Rad2/1 -> Mux/3
  Deg-->Rad3/1 -> Mux/9
  Deg-->Rad1/1 -> Mux/1
  Trigonometric Function3/1 -> Deg-->Rad3/1
  Constant4/1 -> Mux/8
  Trigonometric Function4/1 -> Mux/7
  Constant1/1 -> Mux/6
  Constant3/1 -> Mux/5
  Constant5/1 -> Mux/4
  Trigonometric Function2/1 -> Deg-->Rad2/1
  Constant2/1 -> Mux/2
  Alpha_Deg/1 -> Deg-->Rad/1
  Trigonometric Function/1 -> Deg-->Rad1/1
  Mux/1 -> Reshape/1
  Reshape/1 -> Product/1
  Deg-->Rad/1 -> Trigonometric Function/1, Trigonometric Function2/1, Trigonometric Function3/1, Trigonometric Function4/1
  Stab_Axis/1 -> Product/2
  Product/1 -> Body_Axis/1

== system AeroLib/Aerodynamics/Aerodynamics_Pioneer/Aero Total/Wind2Stab ==
  Beta_Deg : Inport  Port=1  LatchInput=off
  Wind_Axis : Inport  Port=2  LatchInput=off
  Constant{1..2,4..5} (4 alike) : Constant  Value=0
  Constant3 : Constant
  Deg-->Rad : Gain  Gain=pi/180  SaturateOnIntegerOverflow=on
  Deg-->Rad2 : Gain  Gain=-1  SaturateOnIntegerOverflow=on
  Mux : Mux  Inputs=9
  Product : Product  Multiplication=Matrix(*)  SaturateOnIntegerOverflow=on  InputSameDT=on
  Reshape : simulink3/Signals & Systems/Reshape  OutputDimensionality=Customize  OutputDimensions=[3,3]
  Trigonometric Function : Trigonometry  Operator=cos
  Trigonometric Function2 : Trigonometry
  Trigonometric Function3 : Trigonometry  Operator=cos
  Trigonometric Function4 : Trigonometry
  Stab_Axis : Outport
  wires:
  Product/1 -> Stab_Axis/1
  Reshape/1 -> Product/1
  Wind_Axis/1 -> Product/2
  Deg-->Rad2/1 -> Trigonometric Function2/1
  Deg-->Rad/1 -> Deg-->Rad2/1, Trigonometric Function3/1, Trigonometric Function4/1, Trigonometric Function/1
  Mux/1 -> Reshape/1
  Constant3/1 -> Mux/9
  Constant4/1 -> Mux/8
  Constant1/1 -> Mux/7
  Constant5/1 -> Mux/6
  Trigonometric Function3/1 -> Mux/5
  Trigonometric Function4/1 -> Mux/4
  Constant2/1 -> Mux/3
  Trigonometric Function2/1 -> Mux/2
  Trigonometric Function/1 -> Mux/1
  Beta_Deg/1 -> Deg-->Rad/1

== system AeroLib/Aerodynamics/Aerodynamics_Pioneer/Aero_Coefficients/Drag ==
  AlphaDeg : Inport  Port=1  LatchInput=off
  ElevDeg : Inport  Port=2  LatchInput=off
  Alpha : simulink3/Functions & Tables/PreLook-Up Index Search  bpData=Aero.Alpha.CDCL  searchMode=Binary Search  cacheBpFlag=off  outputFlag=off  extrapMode=Linear Extrapolation  rangeErrorMode=None
  Alpha3 : simulink3/Functions & Tables/PreLook-Up Index Search  bpData=Aero.Alpha.Control  searchMode=Binary Search  cacheBpFlag=off  outputFlag=off  extrapMode=Linear Extrapolation  rangeErrorMode=None
  CD : simulink3/Functions & Tables/Interpolation (n-D) using PreLook-Up  numDimsPopupSelect=1  explicitNumDims=2  table=Aero.CD.Total  interpMethod=Linear  extrapMethod=Linear  rangeErrorMode=None
  CD_Elev : simulink3/Functions & Tables/Interpolation (n-D) using PreLook-Up  numDimsPopupSelect=2  explicitNumDims=2  table=Aero.CD.Elev'  interpMethod=Linear  extrapMethod=Linear  rangeErrorMode=None
  Elev : simulink3/Functions & Tables/PreLook-Up Index Search  bpData=Aero.Elev  searchMode=Binary Search  cacheBpFlag=off  outputFlag=off  extrapMode=Linear Extrapolation  rangeErrorMode=None
  Sum : Sum  Inputs=|++  SaturateOnIntegerOverflow=on  InputSameDT=on
  CD_Total : Outport
  wires:
  Sum/1 -> CD_Total/1
  CD_Elev/1 -> Sum/2
  CD/1 -> Sum/1
  ElevDeg/1 -> Elev/1
  AlphaDeg/1 -> Alpha3/1, Alpha/1
  Elev/1 -> CD_Elev/2
  Alpha3/1 -> CD_Elev/1
  Alpha/1 -> CD/1

== system AeroLib/Aerodynamics/Aerodynamics_Pioneer/Aero_Coefficients/Lift ==
  AlphaDeg : Inport  Port=1  LatchInput=off
  ElevDeg : Inport  Port=2  LatchInput=off
  Alpha1 : simulink3/Functions & Tables/PreLook-Up Index Search  bpData=Aero.Alpha.CDCL  searchMode=Binary Search  cacheBpFlag=off  outputFlag=off  extrapMode=Linear Extrapolation  rangeErrorMode=None
  Alpha4 : simulink3/Functions & Tables/PreLook-Up Index Search  bpData=Aero.Alpha.Control  searchMode=Binary Search  cacheBpFlag=off  outputFlag=off  extrapMode=Linear Extrapolation  rangeErrorMode=None
  CL : simulink3/Functions & Tables/Interpolation (n-D) using PreLook-Up  numDimsPopupSelect=1  explicitNumDims=2  table=Aero.CL.Total  interpMethod=Linear  extrapMethod=Linear  rangeErrorMode=None
  CL_Elev : simulink3/Functions & Tables/Interpolation (n-D) using PreLook-Up  numDimsPopupSelect=2  explicitNumDims=2  table=Aero.CL.Elev'  interpMethod=Linear  extrapMethod=Linear  rangeErrorMode=None
  Elev1 : simulink3/Functions & Tables/PreLook-Up Index Search  bpData=Aero.Elev  searchMode=Binary Search  cacheBpFlag=off  outputFlag=off  extrapMode=Linear Extrapolation  rangeErrorMode=None
  Sum : Sum  Inputs=|++  SaturateOnIntegerOverflow=on  InputSameDT=on
  CL_Total : Outport
  wires:
  Sum/1 -> CL_Total/1
  CL_Elev/1 -> Sum/2
  CL/1 -> Sum/1
  ElevDeg/1 -> Elev1/1
  AlphaDeg/1 -> Alpha4/1, Alpha1/1
  Alpha4/1 -> CL_Elev/1
  Elev1/1 -> CL_Elev/2
  Alpha1/1 -> CL/1

== system AeroLib/Aerodynamics/Aerodynamics_Pioneer/Aero_Coefficients/Pitch ==
  AlphaDeg : Inport  Port=1  LatchInput=off
  ElevDeg : Inport  Port=2  LatchInput=off
  Alpha : simulink3/Functions & Tables/PreLook-Up Index Search  bpData=Aero.AlphaCM  searchMode=Binary Search  cacheBpFlag=off  outputFlag=off  extrapMode=Linear Extrapolation  rangeErrorMode=None
  CM_Elev : simulink3/Functions & Tables/Interpolation (n-D) using PreLook-Up  numDimsPopupSelect=2  explicitNumDims=2  table=Aero.CM.Elev'  interpMethod=Linear  extrapMethod=Linear  rangeErrorMode=None
  Elev : simulink3/Functions & Tables/PreLook-Up Index Search  bpData=Aero.ElevCM  searchMode=Binary Search  cacheBpFlag=off  outputFlag=off  extrapMode=Linear Extrapolation  rangeErrorMode=None
  CM_Total : Outport
  wires:
  CM_Elev/1 -> CM_Total/1
  ElevDeg/1 -> Elev/1
  AlphaDeg/1 -> Alpha/1
  Alpha/1 -> CM_Elev/1
  Elev/1 -> CM_Elev/2

== system AeroLib/Aerodynamics/Aerodynamics_Pioneer/Aero_Coefficients/Roll ==
  AlphaDeg : Inport  Port=1  LatchInput=off
  BetaDeg : Inport  Port=2  LatchInput=off
  AilDeg : Inport  Port=3  LatchInput=off
  Ail : simulink/Look-Up Tables/PreLook-Up Index Search  bpData=Aero.Ail  searchMode=Binary Search  cacheBpFlag=off  outputFlag=off  extrapMode=Linear Extrapolation  rangeErrorMode=None
  Alpha : simulink/Look-Up Tables/PreLook-Up Index Search  bpData=Aero.AlphaAil  searchMode=Binary Search  cacheBpFlag=off  outputFlag=off  extrapMode=Linear Extrapolation  rangeErrorMode=None
  CR_Ail : simulink/Look-Up Tables/Interpolation (n-D) using PreLook-Up  numDimsPopupSelect=2  explicitNumDims=2  table=Aero.CR.Ail'  interpMethod=Linear  extrapMethod=Linear  rangeErrorMode=None
  Gain : Gain  Gain=Aero.CR.Beta  SaturateOnIntegerOverflow=on
  Sum : Sum  Inputs=|++  SaturateOnIntegerOverflow=on  InputSameDT=on
  CR_Total : Outport
  wires:
  Sum/1 -> CR_Total/1
  CR_Ail/1 -> Sum/1
  Gain/1 -> Sum/2
  BetaDeg/1 -> Gain/1
  Ail/1 -> CR_Ail/2
  Alpha/1 -> CR_Ail/1
  AlphaDeg/1 -> Alpha/1
  AilDeg/1 -> Ail/1

== system AeroLib/Aerodynamics/Aerodynamics_Pioneer/Aero_Coefficients/SideForce ==
  BetaDeg : Inport  Port=1  LatchInput=off
  RudDeg : Inport  Port=2  LatchInput=off
  AilDeg : Inport  Port=3  LatchInput=off
  Beta : simulink3/Functions & Tables/PreLook-Up Index Search  bpData=Aero.Beta  searchMode=Binary Search  cacheBpFlag=off  outputFlag=off  extrapMode=Linear Extrapolation  rangeErrorMode=None
  CY_Rud : simulink3/Functions & Tables/Interpolation (n-D) using PreLook-Up  numDimsPopupSelect=2  explicitNumDims=2  table=Aero.CY.Rudder'  interpMethod=Linear  extrapMethod=Linear  rangeErrorMode=None
  Deg-->Rad : Gain  Gain=pi/180  SaturateOnIntegerOverflow=on
  Gain1 : Gain  Gain=Aero.CY.Ail  SaturateOnIntegerOverflow=on
  Rudder : simulink3/Functions & Tables/PreLook-Up Index Search  bpData=Aero.Rudder  searchMode=Binary Search  cacheBpFlag=off  outputFlag=off  extrapMode=Linear Extrapolation  rangeErrorMode=None
  Sum : Sum  SaturateOnIntegerOverflow=on  InputSameDT=on
  CY_Total : Outport
  wires:
  Deg-->Rad/1 -> Gain1/1
  Gain1/1 -> Sum/2
  AilDeg/1 -> Deg-->Rad/1
  CY_Rud/1 -> Sum/1
  RudDeg/1 -> Rudder/1
  BetaDeg/1 -> Beta/1
  Beta/1 -> CY_Rud/1
  Rudder/1 -> CY_Rud/2
  Sum/1 -> CY_Total/1

== system AeroLib/Aerodynamics/Aerodynamics_Pioneer/Aero_Coefficients/Yaw ==
  AlphaDeg : Inport  Port=1  LatchInput=off
  BetaDeg : Inport  Port=2  LatchInput=off
  AilDeg : Inport  Port=3  LatchInput=off
  RudDeg : Inport  Port=4  LatchInput=off
  Ail : simulink3/Functions & Tables/PreLook-Up Index Search  bpData=Aero.Ail  searchMode=Binary Search  cacheBpFlag=off  outputFlag=off  extrapMode=Linear Extrapolation  rangeErrorMode=None
  Alpha : simulink3/Functions & Tables/PreLook-Up Index Search  bpData=Aero.Alpha.CDCL  searchMode=Binary Search  cacheBpFlag=off  outputFlag=off  extrapMode=Linear Extrapolation  rangeErrorMode=None
  Beta : simulink3/Functions & Tables/PreLook-Up Index Search  bpData=Aero.BetaCN  searchMode=Binary Search  cacheBpFlag=off  outputFlag=off  extrapMode=Linear Extrapolation  rangeErrorMode=None
  CN_Ail : simulink3/Functions & Tables/Interpolation (n-D) using PreLook-Up  numDimsPopupSelect=2  explicitNumDims=2  table=Aero.CN.Ail'  interpMethod=Linear  extrapMethod=Linear  rangeErrorMode=None
  CN_Rud : simulink3/Functions & Tables/Interpolation (n-D) using PreLook-Up  numDimsPopupSelect=2  explicitNumDims=2  table=Aero.CN.Rudder'  interpMethod=Linear  extrapMethod=Linear  rangeErrorMode=None
  Rud : simulink3/Functions & Tables/PreLook-Up Index Search  bpData=Aero.RudderCN  searchMode=Binary Search  cacheBpFlag=off  outputFlag=off  extrapMode=Linear Extrapolation  rangeErrorMode=None
  Sum : Sum  Inputs=|++  SaturateOnIntegerOverflow=on  InputSameDT=on
  CN_Total : Outport
  wires:
  Beta/1 -> CN_Rud/1
  Rud/1 -> CN_Rud/2
  CN_Ail/1 -> Sum/2
  AilDeg/1 -> Ail/1
  AlphaDeg/1 -> Alpha/1
  Ail/1 -> CN_Ail/2
  Alpha/1 -> CN_Ail/1
  Sum/1 -> CN_Total/1
  CN_Rud/1 -> Sum/1
  RudDeg/1 -> Rud/1
  BetaDeg/1 -> Beta/1

== system AeroLib/Aerodynamics/Aerodynamics_Pioneer/Aero_Dynamic_Coefficients/Aero LatDyn_Coef ==
  p_hat : Inport  Port=1  LatchInput=off
  r_hat : Inport  Port=2  LatchInput=off
  DynCoef Roll_Rate (4) : Subsystem
  DynCoef Yaw_Rate : Subsystem
  Sum : Sum  Inputs=|++  SaturateOnIntegerOverflow=on  InputSameDT=on
  Sum1 : Sum  Inputs=|++  SaturateOnIntegerOverflow=on  InputSameDT=on
  Sum2 : Sum  Inputs=|++  SaturateOnIntegerOverflow=on  InputSameDT=on
  CYdyn : Outport
  CRdyn : Outport  Port=2
  CNdyn : Outport  Port=3
  wires:
  DynCoef Yaw_Rate/3(CNr) -> Sum2/2
  Sum1/1 -> CRdyn/1  "CRp"
  Sum2/1 -> CNdyn/1  "CNp"
  DynCoef Roll_Rate (4)/3(CNp) -> Sum2/1
  DynCoef Roll_Rate (4)/2(CRp) -> Sum1/1
  DynCoef Roll_Rate (4)/1(CYp) -> Sum/1
  Sum/1 -> CYdyn/1
  p_hat/1 -> DynCoef Roll_Rate (4)/1(p_hat)
  r_hat/1 -> DynCoef Yaw_Rate/1(r_hat)
  DynCoef Yaw_Rate/2(CRr) -> Sum1/2
  DynCoef Yaw_Rate/1(CYr) -> Sum/2

== system AeroLib/Aerodynamics/Aerodynamics_Pioneer/Aero_Dynamic_Coefficients/Aero LongDyn_Coef ==
  adot_hat : Inport  Port=1  LatchInput=off
  q_hat : Inport  Port=2  LatchInput=off
  Constant : Constant  Value=0
  Constant1 : Constant  Value=Aero.CL.Alphadot
  Constant2 : Constant  Value=Aero.CL.Qrate
  Constant3 : Constant  Value=Aero.CM.Alphadot
  Constant4 : Constant  Value=Aero.CM.Qrate
  Product{1,4..6} (4 alike) : Product  SaturateOnIntegerOverflow=on  InputSameDT=on
  Sum : Sum  Inputs=+|+  SaturateOnIntegerOverflow=on  InputSameDT=on
  Sum1 : Sum  Inputs=+|+  SaturateOnIntegerOverflow=on  InputSameDT=on
  CDdyn : Outport
  CLdyn : Outport  Port=2
  CMdyn : Outport  Port=3
  wires:
  Sum/1 -> CLdyn/1
  Sum1/1 -> CMdyn/1
  Constant/1 -> CDdyn/1
  Constant1/1 -> Product1/1
  adot_hat/1 -> Product1/2, Product5/2
  Constant2/1 -> Product4/1
  Constant4/1 -> Product6/1
  Constant3/1 -> Product5/1
  q_hat/1 -> Product6/2, Product4/2
  Product5/1 -> Sum1/1
  Product6/1 -> Sum1/2
  Product1/1 -> Sum/1
  Product4/1 -> Sum/2

== system AeroLib/AtmosphericData/AtmosphericData_FAA_gust/Airspeeds/BetaVT ==
  TAS : Inport  Port=1  LatchInput=off
  Beta : Inport  Port=2  LatchInput=off
  BetaVTail : Integrator
  Fcn1 : Fcn  Expr=Geom.Wing.bref*Geom.Vtail.xacvt / u
  FlightTrim_Switch : AeroLib/AMS_StatelessFilters/FlightTrim_Switch
  Product : Product  Inputs=/*  SaturateOnIntegerOverflow=on  InputSameDT=on
  Sum : Sum  Inputs=|+-  SaturateOnIntegerOverflow=on  InputSameDT=on
  BetaVt : Outport
  wires:
  BetaVTail/1 -> BetaVt/1, Sum/2
  Product/1 -> BetaVTail/1
  Fcn1/1 -> Product/1  "tau"
  TAS/1 -> Fcn1/1
  Beta/1 -> Sum/1
  FlightTrim_Switch/1 -> Product/2
  Sum/1 -> FlightTrim_Switch/1  "error"

== system AeroLib/AtmosphericData/AtmosphericData_FAA_gust/Airspeeds/Derivative ==
  Alpha : Inport  Port=1  LatchInput=off
  AlphaDot : Integrator  Orientation=left
  FlightTrim_Switch : AeroLib/AMS_StatelessFilters/FlightTrim_Switch
  Gain : Gain  Gain=20  SaturateOnIntegerOverflow=on
  Sum : Sum  Inputs=|+-  SaturateOnIntegerOverflow=on  InputSameDT=on
  deg_to_rad : Gain  Gain=pi/180  SaturateOnIntegerOverflow=on
  AlphaDot_rad : Outport
  wires:
  Alpha/1 -> Sum/1
  Gain/1 -> AlphaDot/1, deg_to_rad/1
  AlphaDot/1 -> Sum/2
  deg_to_rad/1 -> AlphaDot_rad/1
  FlightTrim_Switch/1 -> Gain/1
  Sum/1 -> FlightTrim_Switch/1

== system AeroLib/AtmosphericData/AtmosphericData_FAA_gust/Airspeeds/Subsystem ==
  Vb : Inport  Port=1  LatchInput=off
  DCM : Inport  Port=2  LatchInput=off
  Wind : Inport  Port=3  LatchInput=off
  Min_TAS : Constant  Value=0.01
  Mod_Va : Fcn  Expr=sqrt(u(1)*u(1)+u(2)*u(2)+u(3)*u(3))
  Sum : Sum  Inputs=|++  SaturateOnIntegerOverflow=on  InputSameDT=on
  Wind_B : Product  Multiplication=Matrix(*)  SaturateOnIntegerOverflow=on  InputSameDT=on
  tas : MinMax  Function=max  Inputs=2  SaturateOnIntegerOverflow=on  InputSameDT=on
  Va : Outport
  TAS : Outport  Port=2
  wires:
  Wind/1 -> Wind_B/2
  DCM/1 -> Wind_B/1
  tas/1 -> TAS/1
  Vb/1 -> Sum/1
  Wind_B/1 -> Sum/2
  Sum/1 -> Va/1, Mod_Va/1
  Mod_Va/1 -> tas/1
  Min_TAS/1 -> tas/2

== system AeroLib/AtmosphericData/FAA_Std_Gust/Turbulence U/Filter_U1 ==
  Noise : Inport  Port=1  LatchInput=off
  Freq : Inport  Port=2  LatchInput=off
  From_Reset : Inport  Port=3  LatchInput=off
  Constant : Constant  Value=0
  Stateless_Integrator : AeroLib/AMS_StatelessFilters/Stateless_Integrator
  Sum : Sum  Inputs=|+-  SaturateOnIntegerOverflow=on  InputSameDT=on
  err_freq : Product  SaturateOnIntegerOverflow=on  InputSameDT=on
  FiltNoise : Outport
  wires:
  Stateless_Integrator/1 -> Sum/2, FiltNoise/1
  Noise/1 -> Sum/1  "noise_u"
  Sum/1 -> err_freq/2  "err"
  Freq/1 -> err_freq/1
  err_freq/1 -> Stateless_Integrator/3
  Constant/1 -> Stateless_Integrator/2
  From_Reset/1 -> Stateless_Integrator/1
